simulink model "Snake_Robot1"  (R2023a)
settings: Solver=VariableStepAuto  StartTime=0.0  StopTime=100  RelTol=1e-5  AbsTol=1e-5
settings Model: Creator=Bhavik  LastModifiedBy=ankitgurjar5494
settings SolverCC: ZeroCrossAlgorithm=Adaptive
settings DataIOCC: ReturnWorkspaceOutputs=off
settings OptimizationCC: ReuseModelBlockBuffer=off

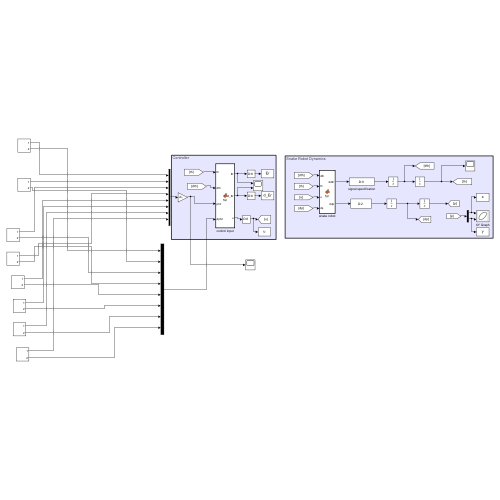
[thumbnail: Simulink's stored preview of the top-level diagram]
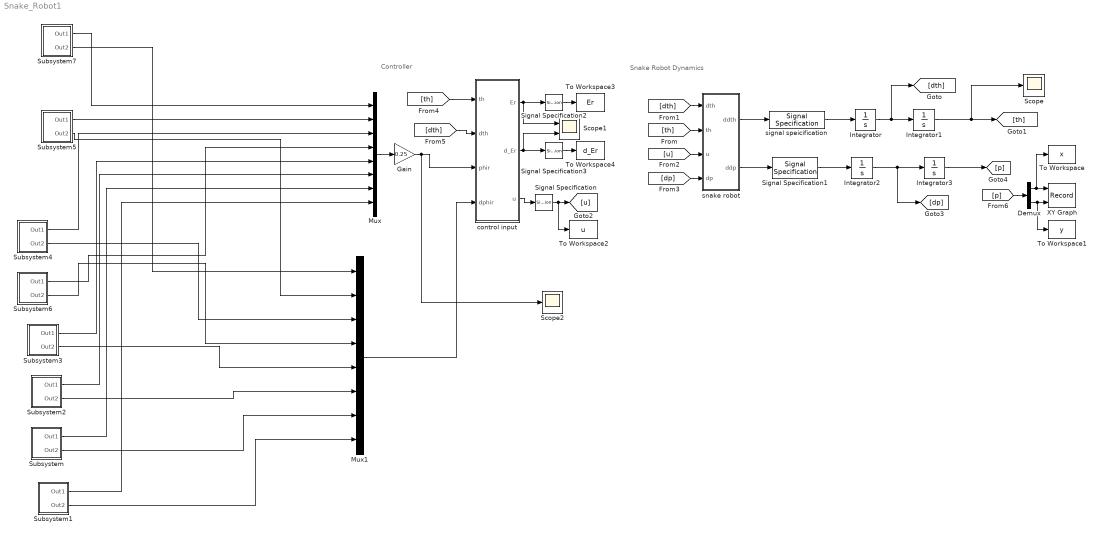
== system Snake_Robot1 ==
  note: Snake Robot Dynamics
  note: Controller
  Demux : Demux  Outputs=2
  Gain : Gain  Gain=0.25
  Integrator{,1..3} (4 alike) : Integrator
  Mux : Mux  Inputs=8
  Mux1 : Mux  Inputs=8
  Scope : Scope
  Scope1 : Scope  NumInputPorts=2
  Scope2 : Scope
  Signal Specification : SignalSpecification  Dimensions=8
  Signal Specification1 : SignalSpecification  Dimensions=2
  Signal Specification2 : SignalSpecification  Dimensions=8
  Signal Specification3 : SignalSpecification  Dimensions=8
  Subsystem : Subsystem
  Subsystem1 : Subsystem
  Subsystem2 : Subsystem
  Subsystem3 : Subsystem
  Subsystem4 : Subsystem
  Subsystem5 : Subsystem
  Subsystem6 : Subsystem
  Subsystem7 : Subsystem
  To Workspace : ToWorkspace  VariableName=x  SampleTime=0.01
  To Workspace1 : ToWorkspace  VariableName=y  SampleTime=0.01
  To Workspace2 : ToWorkspace  VariableName=u  SampleTime=0.01
  To Workspace3 : ToWorkspace  VariableName=Er  SampleTime=0.01
  To Workspace4 : ToWorkspace  VariableName=d_Er  SampleTime=0.01
  XY Graph : Record  FileSettingsInternal="{\"entries\":[{\"content\":{\"excelSettings\":{\"content\":{},\"type\":\"Streamout.ExcelSettings\"}},\"type\":\"Streamout.FileSettingStorage\",\"uuid\":\"c32b7eaa-5569-4195-9e52-34d0314e0fbc\"}],\"packageUris\":[\"http://schema.mathworks.com/mf0/streamout_blocks/R2020a\"],\"version\":\"1.0\"}"  Layout=[1 1]  SignalsInternal="{\"entries\":[{\"content\":{\"signals\":[{\"content\":{\"blockPath\":[\"Snake_Robot1/XY Graph\"],\"dimensions\":[1],\"domain\":\"Snake_Robot1/XY Graph\",\"lineColor\":\"#a2142f\",\"plots\":[1],\"port\":1,\"sid\":[\"\"],\"signalID\":36,\"signalName\":\"Demux:1\"},\"type\":\"RecordBlkView.Signal\",\"uuid\":\"15c8a379-e681-4f2d-87e5-26fa3fdfda9f\"},{\"content\":{\"blockPath\":[\"Snake_Robot1/XY Graph\"],\"dimensions\":[1],\"domain\":\"Snake_Robot1/XY Graph\",\"lineColor\":\"#139fff\",\"plots\":[1],\"port\":2,\"sid\":[\"\"],\"signalID\":40,\"signalName\":\"Demux:2\"},\"type\":\"RecordBlkView.Signal\",\"uuid\":\"109eeb49-de7a-4fca-9ee5-c5d713a50254\"}]},\"type\":\"RecordBlkView.InputSignals\",\"uuid\":\"6f049c98-91aa-4d49-bb40-e600c2961993\"}],\"packageUris\":[\"http://schema.mathworks.com/mf0/streamout_blocks/R2020a\"],\"version\":\"1.0\"}"  VisualizationBindings="{\"xyplotplugin\":{\"info\":[{\"series\":[{\"bindingParametersList\":[{\"parameter\":\"X-Axis\",\"signalID\":36,\"signalName\":\"Demux:1\"},{\"parameter\":\"Y-Axis\",\"signalID\":40,\"signalName\":\"Demux:2\"}],\"seriesID\":50259}],\"subplotID\":1}]}}"  CompatibilityTag=XY
  control input : MATLAB Function  TreatAsAtomicUnit=on
  signal speicification : SignalSpecification  Dimensions=9
  snake robot : MATLAB Function  TreatAsAtomicUnit=on
  wires:
  snake robot/1(ddth) -> signal speicification/1
  snake robot/2(ddp) -> Signal Specification1/1
  signal speicification/1 -> Integrator/1
  Integrator/1 -> [dth], Integrator1/1
  Integrator1/1 -> Scope/1, [th]
  [th] -> snake robot/2(th)
  [dth] -> snake robot/1(dth)
  control input/3(u) -> Signal Specification/1
  [u] -> snake robot/3(u)
  Integrator2/1 -> [dp], Integrator3/1
  Signal Specification1/1 -> Integrator2/1
  Integrator3/1 -> [p]
  [dp] -> snake robot/4(dp)
  [th] -> control input/1(th)
  [dth] -> control input/2(dth)
  Mux/1 -> Gain/1
  Mux1/1 -> control input/4(dphir)
  Demux/2 -> To Workspace1/1, XY Graph/2
  Demux/1 -> To Workspace/1, XY Graph/1
  [p] -> Demux/1
  Signal Specification/1 -> [u], To Workspace2/1
  control input/1(Er) -> Signal Specification2/1, Scope1/1
  control input/2(d_Er) -> Signal Specification3/1, Scope1/2
  Signal Specification2/1 -> To Workspace3/1
  Signal Specification3/1 -> To Workspace4/1
  Subsystem/1(Out1) -> Mux/7
  Subsystem/2(Out2) -> Mux1/7
  Subsystem1/1(Out1) -> Mux/8
  Subsystem1/2(Out2) -> Mux1/8
  Subsystem2/2(Out2) -> Mux1/6
  Subsystem3/2(Out2) -> Mux1/5
  Subsystem4/2(Out2) -> Mux1/3
  Subsystem6/2(Out2) -> Mux1/4
  Subsystem7/2(Out2) -> Mux1/1
  Subsystem7/1(Out1) -> Mux/1
  Subsystem5/1(Out1) -> Mux/2
  Subsystem4/1(Out1) -> Mux/3
  Subsystem6/1(Out1) -> Mux/4
  Subsystem3/1(Out1) -> Mux/5
  Subsystem2/1(Out1) -> Mux/6
  Subsystem5/2(Out2) -> Mux1/2
  Gain/1 -> Scope2/1, control input/3(phir)

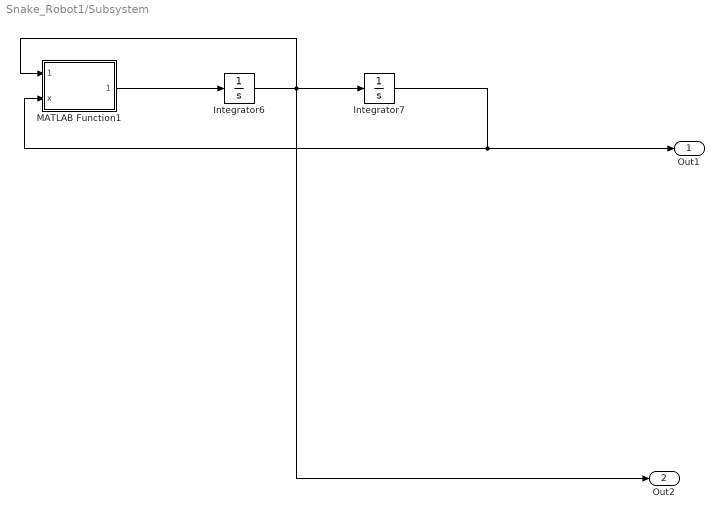
== system Snake_Robot1/Subsystem ==
  Integrator6 : Integrator  InitialCondition=0.1
  Integrator7 : Integrator  InitialCondition=pi/3
  MATLAB Function1 : MATLAB Function  TreatAsAtomicUnit=on
  Out1 : Outport
  Out2 : Outport  Port=2
  wires:
  Integrator7/1 -> Out1/1, MATLAB Function1/2(x)
  Integrator6/1 -> Out2/1, Integrator7/1, MATLAB Function1/1(xprime)
  MATLAB Function1/1(xdoubleprime) -> Integrator6/1

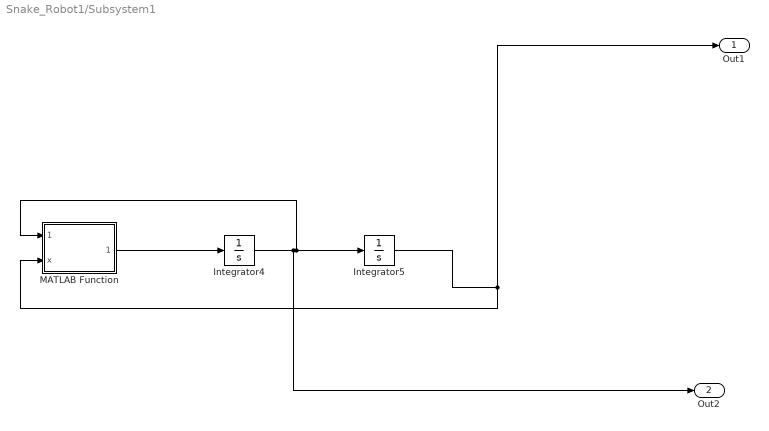
== system Snake_Robot1/Subsystem1 ==
  Integrator4 : Integrator  InitialCondition=0.1
  Integrator5 : Integrator
  MATLAB Function : MATLAB Function  TreatAsAtomicUnit=on
  Out1 : Outport
  Out2 : Outport  Port=2
  wires:
  MATLAB Function/1(xdoubleprime) -> Integrator4/1
  Integrator4/1 -> Out2/1, MATLAB Function/1(xprime), Integrator5/1
  Integrator5/1 -> Out1/1, MATLAB Function/2(x)

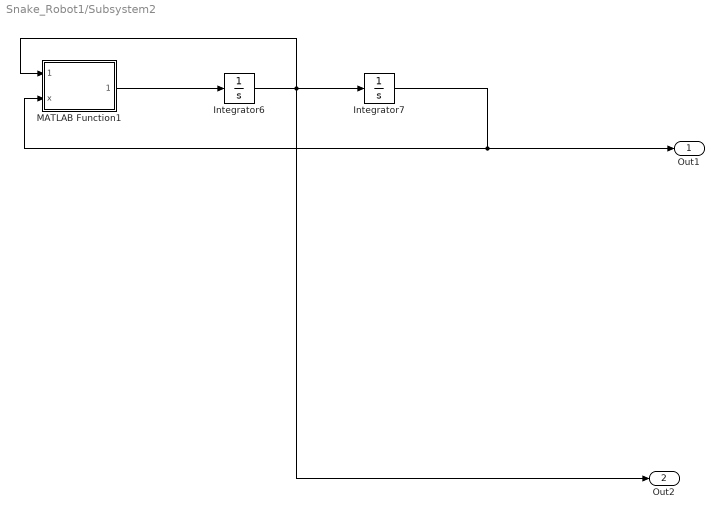
== system Snake_Robot1/Subsystem2 ==
  Integrator6 : Integrator  InitialCondition=0.1
  Integrator7 : Integrator  InitialCondition=2*pi/3
  MATLAB Function1 : MATLAB Function  TreatAsAtomicUnit=on
  Out1 : Outport
  Out2 : Outport  Port=2
  wires:
  MATLAB Function1/1(xdoubleprime) -> Integrator6/1
  Integrator6/1 -> MATLAB Function1/1(xprime), Integrator7/1, Out2/1
  Integrator7/1 -> MATLAB Function1/2(x), Out1/1

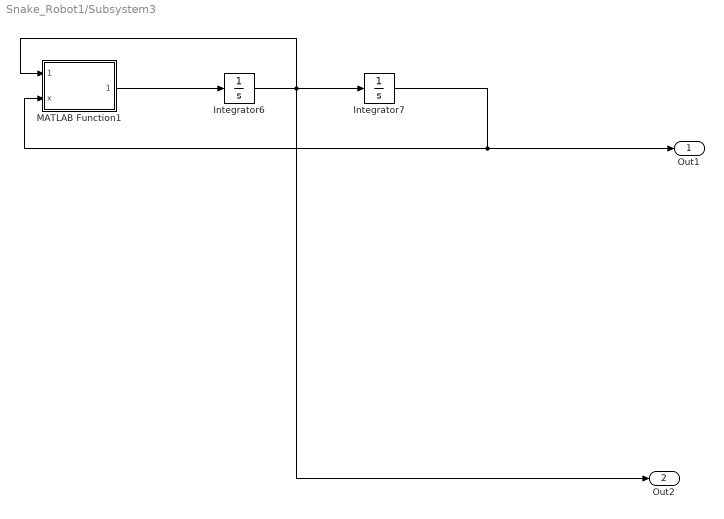
== system Snake_Robot1/Subsystem3 ==
  Integrator6 : Integrator  InitialCondition=0.1
  Integrator7 : Integrator  InitialCondition=3*pi/3
  MATLAB Function1 : MATLAB Function  TreatAsAtomicUnit=on
  Out1 : Outport
  Out2 : Outport  Port=2
  wires:
  Integrator7/1 -> Out1/1, MATLAB Function1/2(x)
  Integrator6/1 -> Out2/1, Integrator7/1, MATLAB Function1/1(xprime)
  MATLAB Function1/1(xdoubleprime) -> Integrator6/1

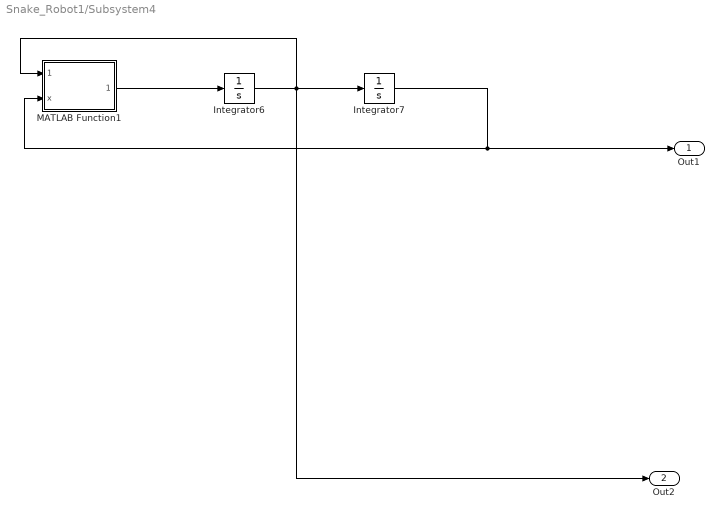
== system Snake_Robot1/Subsystem4 ==
  Integrator6 : Integrator  InitialCondition=0.1
  Integrator7 : Integrator  InitialCondition=5*pi/3
  MATLAB Function1 : MATLAB Function  TreatAsAtomicUnit=on
  Out1 : Outport
  Out2 : Outport  Port=2
  wires:
  MATLAB Function1/1(xdoubleprime) -> Integrator6/1
  Integrator6/1 -> MATLAB Function1/1(xprime), Integrator7/1, Out2/1
  Integrator7/1 -> MATLAB Function1/2(x), Out1/1

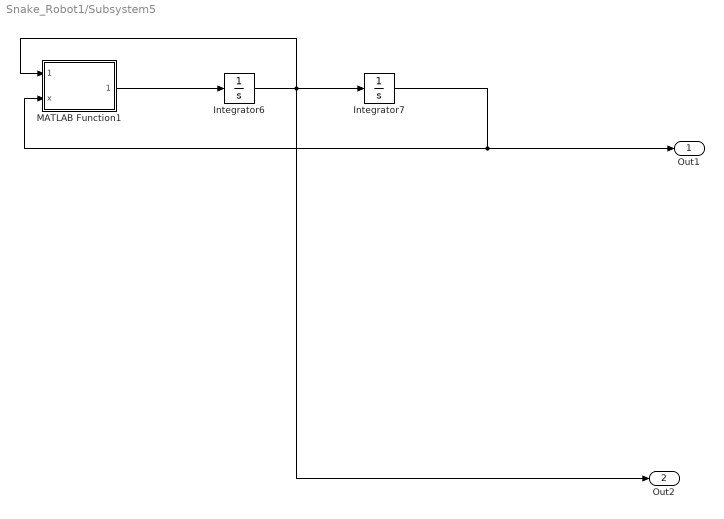
== system Snake_Robot1/Subsystem5 ==
  Integrator6 : Integrator  InitialCondition=0.1
  Integrator7 : Integrator  InitialCondition=6*pi/3
  MATLAB Function1 : MATLAB Function  TreatAsAtomicUnit=on
  Out1 : Outport
  Out2 : Outport  Port=2
  wires:
  Integrator7/1 -> Out1/1, MATLAB Function1/2(x)
  Integrator6/1 -> Out2/1, Integrator7/1, MATLAB Function1/1(xprime)
  MATLAB Function1/1(xdoubleprime) -> Integrator6/1

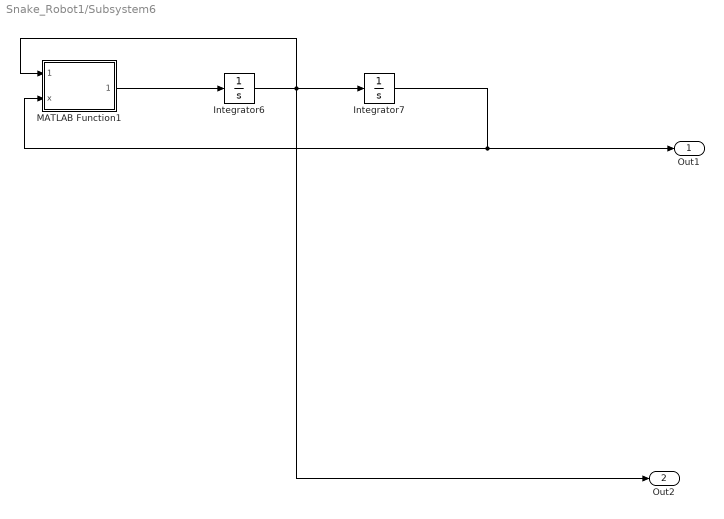
== system Snake_Robot1/Subsystem6 ==
  Integrator6 : Integrator  InitialCondition=0.1
  Integrator7 : Integrator  InitialCondition=4*pi/3
  MATLAB Function1 : MATLAB Function  TreatAsAtomicUnit=on
  Out1 : Outport
  Out2 : Outport  Port=2
  wires:
  MATLAB Function1/1(xdoubleprime) -> Integrator6/1
  Integrator6/1 -> MATLAB Function1/1(xprime), Integrator7/1, Out2/1
  Integrator7/1 -> MATLAB Function1/2(x), Out1/1

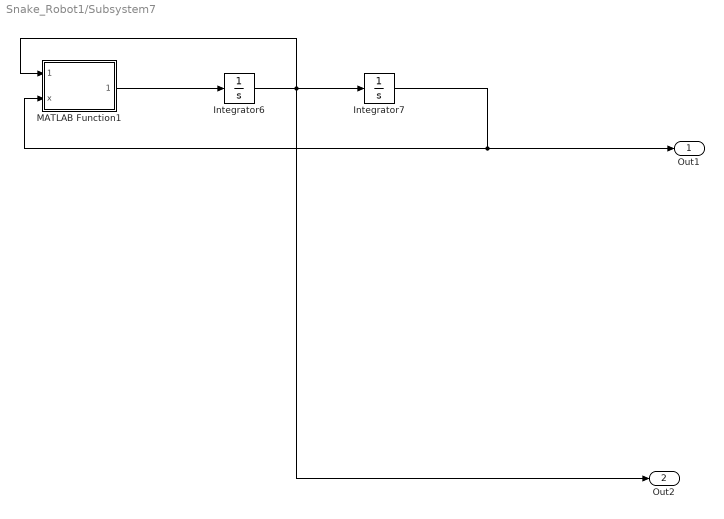
== system Snake_Robot1/Subsystem7 ==
  Integrator6 : Integrator  InitialCondition=0.1
  Integrator7 : Integrator  InitialCondition=7*pi/3
  MATLAB Function1 : MATLAB Function  TreatAsAtomicUnit=on
  Out1 : Outport
  Out2 : Outport  Port=2
  wires:
  Integrator7/1 -> Out1/1, MATLAB Function1/2(x)
  Integrator6/1 -> Out2/1, Integrator7/1, MATLAB Function1/1(xprime)
  MATLAB Function1/1(xdoubleprime) -> Integrator6/1

== matlab function Snake_Robot1/Subsystem6/MATLAB Function1 ==
  data: xprime input; xdoubleprime output; x input
function xdoubleprime = fcn(xprime,x)
% value of coefficient 
xdoubleprime=0.3*(1-x*x)*xprime-x;

== matlab function Snake_Robot1/Subsystem7/MATLAB Function1 ==
  data: xprime input; xdoubleprime output; x input
function xdoubleprime = fcn(xprime,x)
% value of coefficient 
xdoubleprime=0.3*(1-x*x)*xprime-x;

== matlab function Snake_Robot1/Subsystem1/MATLAB Function ==
  data: xprime input; xdoubleprime output; x input
function xdoubleprime = fcn(xprime,x)
% value of coefficient 
xdoubleprime=0.3*(1-x*x)*xprime-x;

== matlab function Snake_Robot1/snake robot ==
  data: dth input; ddth output; th input; ddp output; u input; dp input
function [ddth,ddp] = fcn(dth,th,u,dp)

n = 9; %number of links
m = 0.9047; % mass
l = 0.09; % half link length
J = 1/3*m*l^2; % Mass moment of inertia
ct =2; % tangential drag/friction coefficient
cn =15; % normal drag/friction coefficient
lambda1 = 0.01; % linear torque coefficient
lambda2 = 0.02; % nonlinear torque coefficient

L1 = lambda1*eye(n);
L2 = lambda2*eye(n);

A =[eye(n-1), zeros(n-1,1)]+[zeros(n-1,1),eye(n-1)]; % addition matrix

D = [eye(n-1), zeros(n-1,1)]-[zeros(n-1,1),eye(n-1)]; %substract matrix

e = ones(n,1); %addition vector
E = [e zeros(n,1);zeros(n,1) e];

sinth =zeros(n,1);
costh = zeros(n,1);
for i=1:1:n
sinth(i) = sin(th(i));
costh(i) = cos(th(i));
end

Sth = diag(sinth);
Cth = diag(costh);


V = A'*inv(D*D')*A;
K = A'*inv(D*D')*D;

SCth = [K'*Sth;-K'*Cth];
Mth = J*eye(n) + m*l^2*Sth*V*Sth + m*l^2*Cth*V*Cth; %mass matrix
Wth = m*l^2*Sth*V*Cth - m*l^2*Cth*V*Sth; %coriolis and centripetal matrix
Qth = -[ct*Cth*Cth+cn*Sth*Sth, (ct-cn)*Sth*Cth;
    (ct-cn)*Sth*Cth, ct*Sth*Sth+cn*Cth*Cth];

Fd = l*Qth*SCth*dth + Qth*E*dp; %drag force/friction force

ddth = inv(Mth)*(D'*u - Wth*diag(dth)*dth - L1*dth - L2*diag(abs(dth))*dth + l*SCth'*Fd);
ddp = 1/(n*m)*E'*Fd;

== matlab function Snake_Robot1/Subsystem/MATLAB Function1 ==
  data: xprime input; xdoubleprime output; x input
function xdoubleprime = fcn(xprime,x)
% value of coefficient 
xdoubleprime=0.3*(1-x*x)*xprime-x;

== matlab function Snake_Robot1/Subsystem2/MATLAB Function1 ==
  data: xprime input; xdoubleprime output; x input
function xdoubleprime = fcn(xprime,x)
% value of coefficient 
xdoubleprime=0.3*(1-x*x)*xprime-x;

== matlab function Snake_Robot1/control input ==
  data: Er output; d_Er output; th input; dth input; u output; phir input; dphir input
function [Er,d_Er,u] = fcn(th,dth,phir,dphir)
n = 9; % number of links
D = [eye(n-1), zeros(n-1,1)]-[zeros(n-1,1),eye(n-1)]; %substract matrix
kp = 20; %proportional gain
kd = 5; %derivative gain
Er = D*th-phir; %position error
d_Er = D*dth-dphir; %velocity error
u =-kp*Er-kd*d_Er; %output torque

== matlab function Snake_Robot1/Subsystem3/MATLAB Function1 ==
  data: xprime input; xdoubleprime output; x input
function xdoubleprime = fcn(xprime,x)
% value of coefficient 
xdoubleprime=0.3*(1-x*x)*xprime-x;

== matlab function Snake_Robot1/Subsystem4/MATLAB Function1 ==
  data: xprime input; xdoubleprime output; x input
function xdoubleprime = fcn(xprime,x)
% value of coefficient 
xdoubleprime=0.3*(1-x*x)*xprime-x;

== matlab function Snake_Robot1/Subsystem5/MATLAB Function1 ==
  data: xprime input; xdoubleprime output; x input
function xdoubleprime = fcn(xprime,x)
% value of coefficient 
xdoubleprime=0.3*(1-x*x)*xprime-x;
